simulink model "klf_all"  (R2021a)
settings: Solver=FixedStepAuto  StartTime=0.0  StopTime=10  FixedStep=0.1  RelTol=1e-3
PreLoadFcn:
  | Q = 0.1;
  | R1 = 1;
  | R2 = 0.9;
  | kl = 0;
CloseFcn:
  | clear all
  | try
  | rmdir slprj\ s
  | catch
  | end
  | try
  | folder_name = [bdroot '*'];
  | rmdir(folder_name,'s')
  | catch
  | end
  | try
  | file_temp_name = [bdroot '.slxc'];
  | delete(file_temp_name)
  | %%delete *.mexw64
  | catch
  | end
  | clear folder_name file_temp_name
settings Model: Creator=jetson  LastModifiedBy=jetson
settings DataIOCC: SaveOutput=off  DSMLogging=off  SaveTime=off  ReturnWorkspaceOutputs=off
settings OptimizationCC: DefaultParameterBehavior=Inlined  EnhancedBackFolding=on  PassReuseOutputArgsAs=Individual arguments  ZeroExternalMemoryAtStartup=off  ZeroInternalMemoryAtStartup=off  OptimizeBlockOrder=speed  DifferentSizesBufferReuse=on  OptimizationCustomize=off  EfficientTunableParamExpr=on
settings DebuggingCC: ParameterTunabilityLossMsg=error
settings SFSimCC: MATLABDynamicMemAlloc=off
settings RTWCC: SystemTargetFile=ert.tlc  GenCodeOnly=on  TemplateMakefile=ert_default_tmf  GenerateReport=on  RTWUseSimCustomCode=on  IncludeHyperlinkInReport=on  LaunchReport=on  GenerateTraceInfo=on
settings CodeAppCC: ForceParamTrailComments=on  IgnoreCustomStorageClasses=off  OperatorAnnotations=on  SimulinkDataObjDesc=on  SFDataObjDesc=on  InsertBlockDesc=on
settings ERTTargetCC: TargetLangStandard=C99 (ISO)  GenerateSampleERTMain=on  InlinedParameterPlacement=NonHierarchical  ERTCustomFileTemplate=example_file_process.tlc

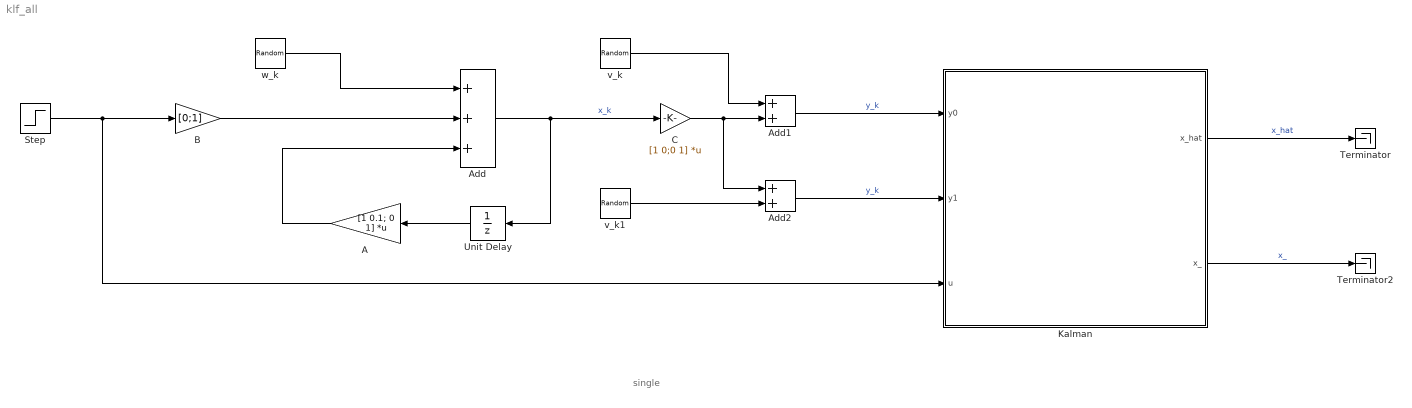
== system klf_all ==
  note: single
  A : Gain  Gain=[1 0.1; 0 1]  Multiplication=Matrix(K*u)
      settings: AttributesFormatString=A = %<Gain>
  Add : Sum  Inputs=3
  Add1 : Sum
  Add2 : Sum
  B : Gain  Gain=[0;1]
      settings: AttributesFormatString=B = %<Gain>
  C : Gain  Gain=[1 0;0 1]  Multiplication=Matrix(K*u)
      settings: AttributesFormatString=C = %<Gain>
  Kalman : Subsystem  Variant=on
  Step : Step  Before=1  After=0
  Terminator : Terminator
  Terminator2 : Terminator
  Unit Delay : UnitDelay  InitialCondition=[0;0]  SampleTime=-1  HasFrameUpgradeWarning=on
  v_k : RandomNumber  Mean=[0; 0]  Variance=[R1; R1]  Seed=[1000; 700]
      settings: AttributesFormatString=|
      | var = %<Variance>
      | mean = %<Mean>
  v_k1 : RandomNumber  Mean=[0; 0]  Variance=[R2; R2]  Seed=[100; 70]
      settings: AttributesFormatString=|
      | var = %<Variance>
      | mean = %<Mean>
  "w_k " : RandomNumber  Mean=[0; 0]  Variance=[Q;Q]  Seed=[3; 100]
      settings: AttributesFormatString=|
      | var = %<Variance>
      | mean = %<Mean>
  wires:
  Unit Delay/1 -> A/1
  Add/1 -> Unit Delay/1, C/1  "x_k"
  A/1 -> Add/3
  B/1 -> Add/2
  Step/1 -> Kalman/3(u), B/1
  v_k/1 -> Add1/1
  C/1 -> Add2/1, Add1/2
  Add1/1 -> Kalman/1(y0)  "y_k"
  "w_k "/1 -> Add/1
  Kalman/1(x_hat) -> Terminator/1  "x_hat"
  Kalman/2(x_) -> Terminator2/1  "x_"
  v_k1/1 -> Add2/2
  Add2/1 -> Kalman/2(y1)  "y_k"

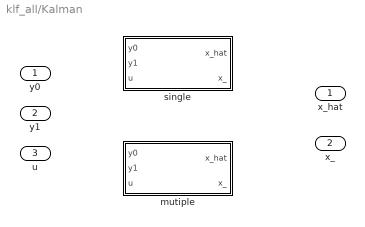
== system klf_all/Kalman ==
  y0 : Inport
  y1 : Inport  Port=2
  u : Inport  Port=3
  mutiple : Subsystem  VariantControl=kl==1
  single : Subsystem  VariantControl=kl==0
  x_hat : Outport
  x_ : Outport  Port=2

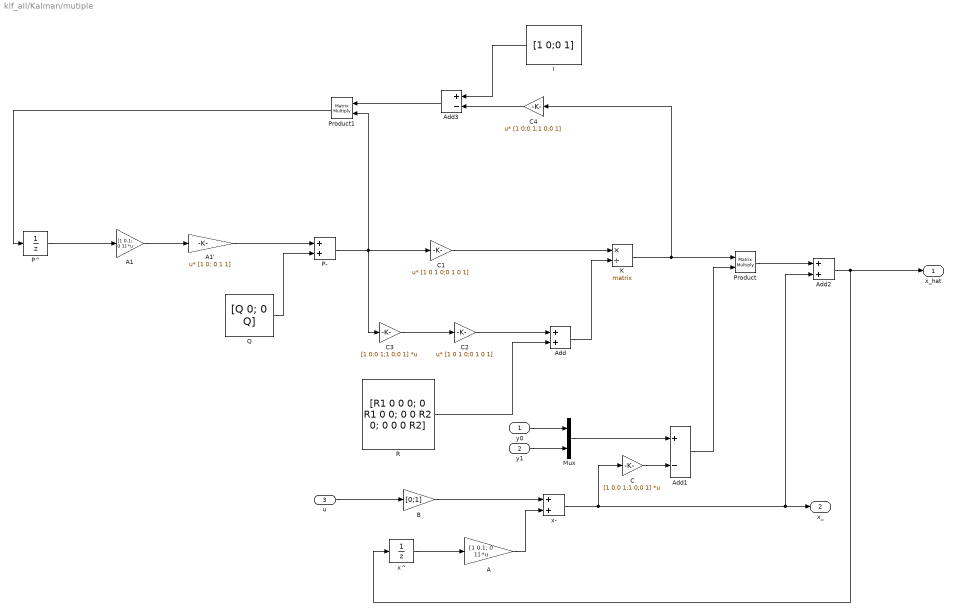
== system klf_all/Kalman/mutiple ==
  y0 : Inport
  y1 : Inport  Port=2
  u : Inport  Port=3
  A : Gain  Gain=[1 0.1; 0 1]  Multiplication=Matrix(K*u)
      settings: AttributesFormatString=A = %<Gain>
  A1 : Gain  Gain=[1 0.1; 0 1]  Multiplication=Matrix(K*u)
      settings: AttributesFormatString=A = %<Gain>
  A1' : Gain  Gain=[1 0; 0.1 1]  Multiplication=Matrix(u*K)
      settings: AttributesFormatString=A = %<Gain>
  Add : Sum
  Add1 : Sum  Inputs=+-
  Add2 : Sum
  Add3 : Sum  Inputs=+-
  B : Gain  Gain=[0;1]
      settings: AttributesFormatString=B = %<Gain>
  C : Gain  Gain=[1 0;0 1;1 0;0 1]  Multiplication=Matrix(K*u)
      settings: AttributesFormatString=C = %<Gain>
  C1 : Gain  Gain=[1 0 1 0;0 1 0 1]  Multiplication=Matrix(u*K)
      settings: AttributesFormatString=C = %<Gain>
  C2 : Gain  Gain=[1 0 1 0;0 1 0 1]  Multiplication=Matrix(u*K)
      settings: AttributesFormatString=C = %<Gain>
  C3 : Gain  Gain=[1 0;0 1;1 0;0 1]  Multiplication=Matrix(K*u)
      settings: AttributesFormatString=C = %<Gain>
  C4 : Gain  Gain=[1 0;0 1;1 0;0 1]  Multiplication=Matrix(u*K)
      settings: AttributesFormatString=C = %<Gain>
  I : Constant  Value=[1 0;0 1]
  K : Product  Inputs=*/  Multiplication=Matrix(*)
  Mux : Mux  Inputs=2
  P- : Sum
  P^ : UnitDelay  InitialCondition=[1 0; 0 1]  SampleTime=-1  HasFrameUpgradeWarning=on
  Product : Product  Multiplication=Matrix(*)
  Product1 : Product  Multiplication=Matrix(*)
  Q : Constant  Value=[Q 0; 0 Q]
  R : Constant  Value=[R1 0 0 0; 0 R1 0 0; 0 0 R2 0; 0 0 0 R2]
  x- : Sum
  x^ : UnitDelay  InitialCondition=[10;10]  SampleTime=-1  HasFrameUpgradeWarning=on
  x_hat : Outport
  x_ : Outport  Port=2
  wires:
  Add1/1 -> Product/2
  R/1 -> Add/2
  C/1 -> Add1/2
  C3/1 -> C2/1
  Product/1 -> Add2/1
  Product1/1 -> P^/1
  x^/1 -> A/1
  Add/1 -> K/2
  Mux/1 -> Add1/1
  y1/1 -> Mux/2
  A/1 -> x-/2
  x-/1 -> C/1, x_/1, Add2/2
  B/1 -> x-/1
  C4/1 -> Add3/2
  Q/1 -> P-/2
  Add2/1 -> x_hat/1, x^/1
  Add3/1 -> Product1/1
  C1/1 -> K/1
  I/1 -> Add3/1
  A1'/1 -> P-/1
  C2/1 -> Add/1
  A1/1 -> A1'/1
  y0/1 -> Mux/1
  P-/1 -> C3/1, Product1/2, C1/1
  K/1 -> C4/1, Product/1
  P^/1 -> A1/1
  u/1 -> B/1

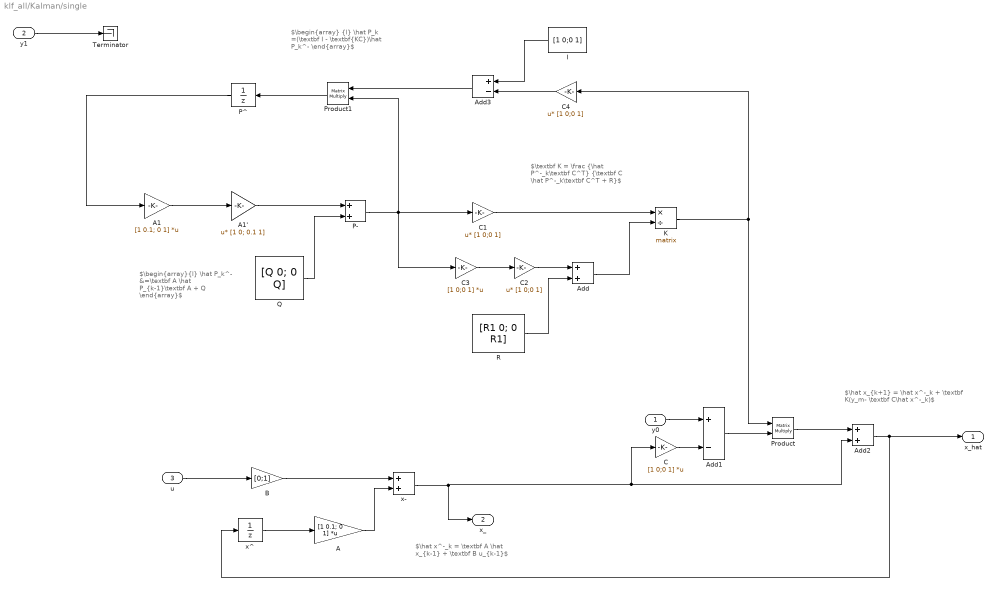
== system klf_all/Kalman/single ==
  note: $\hat x^-_k = \textbf A \hat x_{k-1} + \textbf B u_{k-1}$
  note: $\hat x_{k+1} = \hat x^-_k + \textbf K(y_m- \textbf C\hat x^-_k)$
  note: $\begin{array}{l} \hat P_k^- &=\textbf A \hat P_{k-1}\textbf A + Q \end{array}$
  note: $\begin{array} {l} \hat P_k =(\textbf I - \textbf{KC})\hat P_k^- \end{array}$
  note: $\textbf K = \frac {\hat P^-_k\textbf C^T} {\textbf C \hat P^-_k\textbf C^T + R}$
  y0 : Inport
  y1 : Inport  Port=2
  u : Inport  Port=3
  A : Gain  Gain=[1 0.1; 0 1]  Multiplication=Matrix(K*u)
      settings: AttributesFormatString=A = %<Gain>
  A1 : Gain  Gain=[1 0.1; 0 1]  Multiplication=Matrix(K*u)
      settings: AttributesFormatString=A = %<Gain>
  A1' : Gain  Gain=[1 0; 0.1 1]  Multiplication=Matrix(u*K)
      settings: AttributesFormatString=A = %<Gain>
  Add : Sum
  Add1 : Sum  Inputs=+-
  Add2 : Sum
  Add3 : Sum  Inputs=+-
  B : Gain  Gain=[0;1]
      settings: AttributesFormatString=B = %<Gain>
  C : Gain  Gain=[1 0;0 1]  Multiplication=Matrix(K*u)
      settings: AttributesFormatString=C = %<Gain>
  C1 : Gain  Gain=[1 0;0 1]  Multiplication=Matrix(u*K)
      settings: AttributesFormatString=C = %<Gain>
  C2 : Gain  Gain=[1 0;0 1]  Multiplication=Matrix(u*K)
      settings: AttributesFormatString=C = %<Gain>
  C3 : Gain  Gain=[1 0;0 1]  Multiplication=Matrix(K*u)
      settings: AttributesFormatString=C = %<Gain>
  C4 : Gain  Gain=[1 0;0 1]  Multiplication=Matrix(u*K)
      settings: AttributesFormatString=C = %<Gain>
  I : Constant  Value=[1 0;0 1]
  K : Product  Inputs=*/  Multiplication=Matrix(*)
  P- : Sum
  P^ : UnitDelay  InitialCondition=[1 0; 0 1]  SampleTime=-1  HasFrameUpgradeWarning=on
  Product : Product  Multiplication=Matrix(*)
  Product1 : Product  Multiplication=Matrix(*)
  Q : Constant  Value=[Q 0; 0 Q]
  R : Constant  Value=[R1 0; 0 R1]
  Terminator : Terminator
  x- : Sum
  x^ : UnitDelay  InitialCondition=[0;0]  SampleTime=-1  HasFrameUpgradeWarning=on
      settings: AttributesFormatString=init = %<InitialCondition>
  x_hat : Outport
  x_ : Outport  Port=2
  wires:
  I/1 -> Add3/1
  Add3/1 -> Product1/1
  Add1/1 -> Product/2
  K/1 -> C4/1, Product/1
  C3/1 -> C2/1
  P-/1 -> C1/1, Product1/2, C3/1
  C4/1 -> Add3/2
  Product/1 -> Add2/1
  C2/1 -> Add/1
  Add2/1 -> x_hat/1, x^/1
  A1'/1 -> P-/1
  Q/1 -> P-/2
  P^/1 -> A1/1
  C1/1 -> K/1
  y0/1 -> Add1/1
  Add/1 -> K/2
  C/1 -> Add1/2
  R/1 -> Add/2
  x-/1 -> x_/1, Add2/2, C/1
  A1/1 -> A1'/1
  Product1/1 -> P^/1
  A/1 -> x-/2
  x^/1 -> A/1
  B/1 -> x-/1
  u/1 -> B/1
  y1/1 -> Terminator/1
